simulink model "WG0920_3D"  (R2013a)
settings: Solver=ode3  StartTime=0.0  StopTime=T  FixedStep=dt  RelTol=1e-3
values from neighbouring files (symbols this model uses):
  dt = 1e-2    (= 0.01)    [WGSim.m]
  vi = [0,0,0,0,0,0,0,0,0,0,0,0]    [WGSim.m]
  xi = [0,0,0,0,0,0,0,0,0,0,0,0]    [WGSim.m]
libraries: simulink x2
settings Model: Creator=user  LastModifiedBy=user

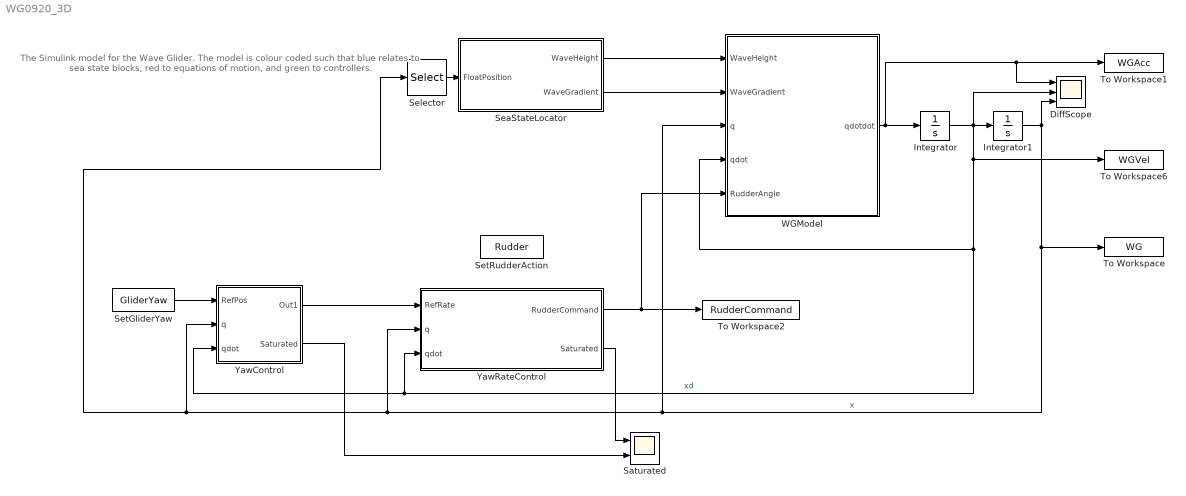
== system WG0920_3D ==
  note: The Simulink model for the Wave Glider.
      | The model is colour coded such that blue
      | relates to sea state blocks, red to equations
      | of motion, and green to controllers.
  DiffScope : Scope  NumInputPorts=3
      settings: ShowLegends=on  TimeRange=10  YMin=-17~-1.1~-2  YMax=5~0.8~4.5
  Integrator : Integrator  InitialCondition=vi  ContinuousStateAttributes='velocity'
  Integrator1 : Integrator  InitialCondition=xi  ContinuousStateAttributes='position'
  Saturated : Scope  NumInputPorts=2
      settings: ShowLegends=on  YMin=-2.75~-2  YMax=2~2  SaveName=ScopeData15
  SeaStateLocator : Subsystem
  Selector : Selector  InputPortWidth=12  IndexOptions=Index vector (dialog)  Indices=[1 2]  OutputSizes=1
  SetGliderYaw : FromWorkspace  VariableName=GliderYaw  SampleTime=0  OutputAfterFinalValue=Holding final value
  SetRudderAction : FromWorkspace  VariableName=Rudder  SampleTime=0  OutputAfterFinalValue=Holding final value
  To Workspace : ToWorkspace  VariableName=WG  SampleTime=-1
  To Workspace1 : ToWorkspace  VariableName=WGAcc  SampleTime=-1
  To Workspace2 : ToWorkspace  VariableName=RudderCommand  SampleTime=-1
  To Workspace6 : ToWorkspace  VariableName=WGVel  SampleTime=-1
  WGModel : Subsystem
  YawControl : Subsystem
  YawRateControl : Subsystem
  wires:
  Integrator/1 -> DiffScope/2, YawControl/3(qdot), YawRateControl/3(qdot), WGModel/4(qdot), To Workspace6/1, Integrator1/1  "xd"
  Integrator1/1 -> DiffScope/3, WGModel/3(q), YawRateControl/2(q), YawControl/2(q), Selector/1, To Workspace/1  "x"
  WGModel/1(qdotdot) -> DiffScope/1, To Workspace1/1, Integrator/1
  Selector/1 -> SeaStateLocator/1(FloatPosition)
  SeaStateLocator/1(WaveHeight) -> WGModel/1(WaveHeight)
  SeaStateLocator/2(WaveGradient) -> WGModel/2(WaveGradient)
  YawRateControl/1(RudderCommand) -> WGModel/5(RudderAngle), To Workspace2/1
  SetGliderYaw/1 -> YawControl/1(RefPos)
  YawControl/1(Out1) -> YawRateControl/1(RefRate)
  YawRateControl/2(Saturated) -> Saturated/1
  YawControl/2(Saturated) -> Saturated/2

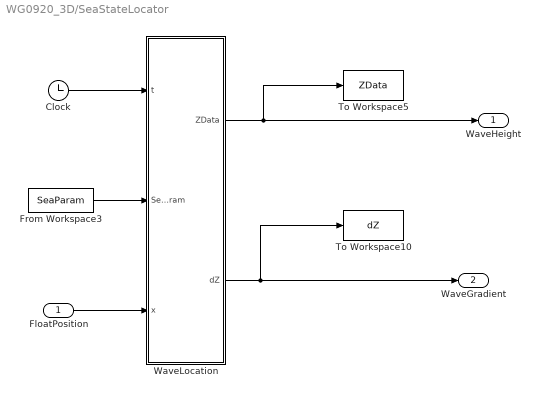
== system WG0920_3D/SeaStateLocator ==
  FloatPosition : Inport
  Clock : Clock
  From Workspace3 : FromWorkspace  VariableName=SeaParam  SampleTime=0  Interpolate=off  OutputAfterFinalValue=Holding final value
  To Workspace10 : ToWorkspace  VariableName=dZ  SampleTime=-1
  To Workspace5 : ToWorkspace  VariableName=ZData  SampleTime=-1
  WaveLocation : MATLAB Function  TreatAsAtomicUnit=on  SystemSampleTime=dt
  WaveHeight : Outport
  WaveGradient : Outport  Port=2
  wires:
  WaveLocation/1(ZData) -> WaveHeight/1, To Workspace5/1
  From Workspace3/1 -> WaveLocation/2(SeaParam)
  WaveLocation/2(dZ) -> To Workspace10/1, WaveGradient/1
  FloatPosition/1 -> WaveLocation/3(x)
  Clock/1 -> WaveLocation/1(t)

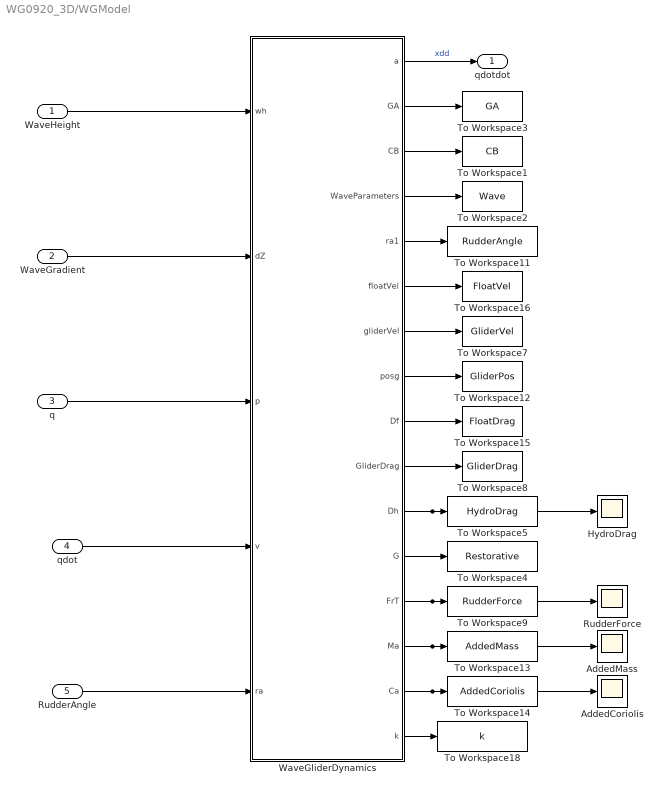
== system WG0920_3D/WGModel ==
  WaveHeight : Inport
  WaveGradient : Inport  Port=2
  q : Inport  Port=3
  qdot : Inport  Port=4
  RudderAngle : Inport  Port=5
  AddedCoriolis : Scope
      settings: ShowLegends=on  SaveName=ScopeData13
  AddedMass : Scope
      settings: ShowLegends=on  SaveName=ScopeData7
  HydroDrag : Scope
      settings: ShowLegends=on
  RudderForce : Scope
      settings: ShowLegends=on  SaveName=ScopeData9
  To Workspace1 : ToWorkspace  VariableName=CB  SampleTime=-1
  To Workspace11 : ToWorkspace  VariableName=RudderAngle  SampleTime=-1
  To Workspace12 : ToWorkspace  VariableName=GliderPos  SampleTime=-1
  To Workspace13 : ToWorkspace  VariableName=AddedMass  SampleTime=-1
  To Workspace14 : ToWorkspace  VariableName=AddedCoriolis  SampleTime=-1
  To Workspace15 : ToWorkspace  VariableName=FloatDrag  SampleTime=-1
  To Workspace16 : ToWorkspace  VariableName=FloatVel  SampleTime=-1
  To Workspace18 : ToWorkspace  VariableName=k  SampleTime=-1
  To Workspace2 : ToWorkspace  VariableName=Wave  SampleTime=-1
  To Workspace3 : ToWorkspace  VariableName=GA  SampleTime=-1
  To Workspace4 : ToWorkspace  VariableName=Restorative  SampleTime=-1
  To Workspace5 : ToWorkspace  VariableName=HydroDrag  SampleTime=-1
  To Workspace7 : ToWorkspace  VariableName=GliderVel  SampleTime=-1
  To Workspace8 : ToWorkspace  VariableName=GliderDrag  SampleTime=-1
  To Workspace9 : ToWorkspace  VariableName=RudderForce  SampleTime=-1
  WaveGliderDynamics : MATLAB Function  TreatAsAtomicUnit=on
  qdotdot : Outport
  wires:
  WaveGliderDynamics/12(G) -> To Workspace4/1
  WaveGliderDynamics/13(FrT) -> RudderForce/1, To Workspace9/1
  WaveGliderDynamics/4(WaveParameters) -> To Workspace2/1
  WaveGradient/1 -> WaveGliderDynamics/2(dZ)
  WaveGliderDynamics/1(a) -> qdotdot/1  "xdd"
  WaveGliderDynamics/10(GliderDrag) -> To Workspace8/1
  WaveGliderDynamics/16(k) -> To Workspace18/1
  WaveGliderDynamics/8(posg) -> To Workspace12/1
  WaveGliderDynamics/9(Df) -> To Workspace15/1
  WaveGliderDynamics/15(Ca) -> AddedCoriolis/1, To Workspace14/1
  WaveHeight/1 -> WaveGliderDynamics/1(wh)
  q/1 -> WaveGliderDynamics/3(p)
  qdot/1 -> WaveGliderDynamics/4(v)
  WaveGliderDynamics/3(CB) -> To Workspace1/1
  WaveGliderDynamics/5(ra1) -> To Workspace11/1
  WaveGliderDynamics/2(GA) -> To Workspace3/1
  RudderAngle/1 -> WaveGliderDynamics/5(ra)
  WaveGliderDynamics/6(floatVel) -> To Workspace16/1
  WaveGliderDynamics/14(Ma) -> AddedMass/1, To Workspace13/1
  WaveGliderDynamics/7(gliderVel) -> To Workspace7/1
  WaveGliderDynamics/11(Dh) -> To Workspace5/1, HydroDrag/1

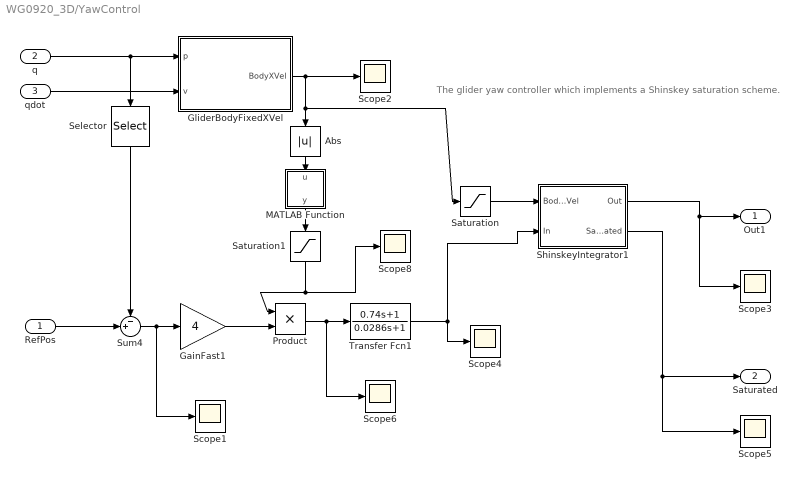
== system WG0920_3D/YawControl ==
  note: The glider yaw controller which implements
      | a Shinskey saturation scheme.
  RefPos : Inport
  q : Inport  Port=2
  qdot : Inport  Port=3
  Abs : Abs
  GainFast1 : Gain  Gain=4
  GliderBodyFixedXVel : MATLAB Function  TreatAsAtomicUnit=on
  MATLAB Function : MATLAB Function  TreatAsAtomicUnit=on
  Product : Product
  Saturation : Saturate  UpperLimit=1.5  LowerLimit=0.1
  Saturation1 : Saturate  UpperLimit=1  LowerLimit=0.01
  Scope{1..6,8} (7 alike) : Scope
      Scope1 settings: YMin=-0.45  YMax=0.2  SaveName=ScopeData10
      Scope2 settings: YMin=-0.2  YMax=0.2  SaveName=ScopeData11
      Scope3 settings: YMin=-0.08  YMax=0.08  SaveName=ScopeData6
      Scope4 settings: YMin=0.01  YMax=0.05  SaveName=ScopeData12
      Scope5 settings: YMin=-0.2  YMax=1.2  SaveName=ScopeData14
      Scope6 settings: YMin=-0.025  YMax=0.25  SaveName=ScopeData17
      Scope8 settings: YMin=-0.025  YMax=0.25  SaveName=ScopeData16
  Selector : Selector  InputPortWidth=12  IndexOptions=Index vector (dialog)  Indices=[11]  OutputSizes=1
  ShinskeyIntegrator1 : Subsystem
  Sum4 : Sum  Inputs=-+|
  Transfer Fcn1 : TransferFcn  Numerator=[0.74 1]  Denominator=[0.0286 1]
  Out1 : Outport
  Saturated : Outport  Port=2
  wires:
  RefPos/1 -> Sum4/2
  q/1 -> GliderBodyFixedXVel/1(p), Selector/1
  Selector/1 -> Sum4/1
  ShinskeyIntegrator1/1(Out) -> Out1/1, Scope3/1
  Transfer Fcn1/1 -> Scope4/1, ShinskeyIntegrator1/2(In)
  qdot/1 -> GliderBodyFixedXVel/2(v)
  Sum4/1 -> Scope1/1, GainFast1/1
  Saturation/1 -> ShinskeyIntegrator1/1(BodyFixedVel)
  ShinskeyIntegrator1/2(Saturated) -> Scope5/1, Saturated/1
  GliderBodyFixedXVel/1(BodyXVel) -> Scope2/1, Abs/1, Saturation/1
  Saturation1/1 -> Scope8/1, Product/1
  Abs/1 -> MATLAB Function/1(u)
  MATLAB Function/1(y) -> Saturation1/1
  GainFast1/1 -> Product/2
  Product/1 -> Transfer Fcn1/1, Scope6/1

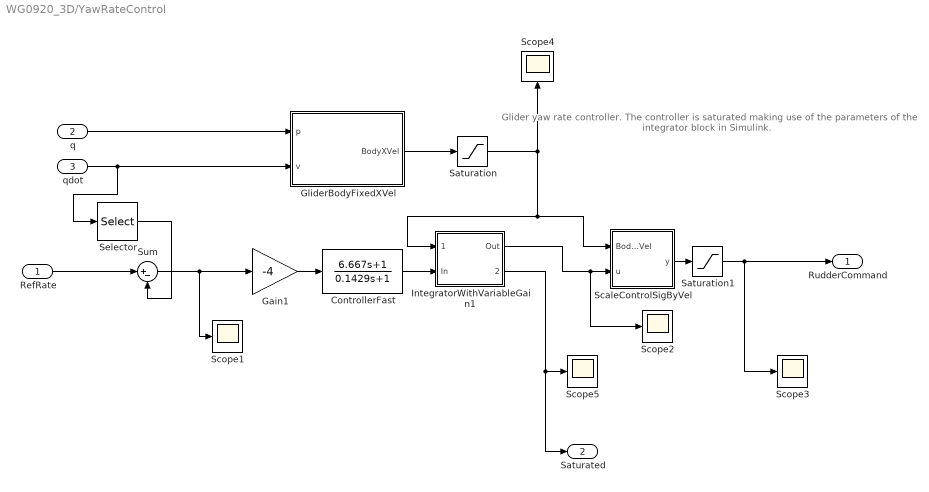
== system WG0920_3D/YawRateControl ==
  note: Glider yaw rate controller. The controller
      | is saturated making use of the parameters
      | of the integrator block in Simulink.
  RefRate : Inport
  q : Inport  Port=2
  qdot : Inport  Port=3
  ControllerFast : TransferFcn  Numerator=[6.667 1]  Denominator=[0.1429 1]
  Gain1 : Gain  Gain=-4
  GliderBodyFixedXVel : MATLAB Function  TreatAsAtomicUnit=on
  IntegratorWithVariableGain1 : Subsystem
  Saturation : Saturate  UpperLimit=1.5  LowerLimit=0.1
  Saturation1 : Saturate  UpperLimit=pi/18*5  LowerLimit=-pi/18*5
  ScaleControlSigByVel : MATLAB Function  TreatAsAtomicUnit=on
  Scope{1..5} (5 alike) : Scope
      Scope1 settings: SaveName=ScopeData3
      Scope2 settings: SaveName=ScopeData4
      Scope3 settings: YMin=0.0665  YMax=0.0681  SaveName=ScopeData5
      Scope4 settings: YMin=-0.00085  YMax=-0.0001  SaveName=ScopeData2
      Scope5 settings: SaveName=ScopeData8
  Selector : Selector  InputPortWidth=12  IndexOptions=Index vector (dialog)  Indices=[11]  OutputSizes=1
  Sum : Sum  Inputs=|+-
  RudderCommand : Outport
  Saturated : Outport  Port=2
  wires:
  ScaleControlSigByVel/1(y) -> Saturation1/1
  Saturation/1 -> ScaleControlSigByVel/1(BodyXVel), IntegratorWithVariableGain1/1(BodyXVel), Scope4/1
  RefRate/1 -> Sum/1
  Sum/1 -> Scope1/1, Gain1/1
  Saturation1/1 -> Scope3/1, RudderCommand/1
  q/1 -> GliderBodyFixedXVel/1(p)
  qdot/1 -> Selector/1, GliderBodyFixedXVel/2(v)
  Selector/1 -> Sum/2
  Gain1/1 -> ControllerFast/1
  GliderBodyFixedXVel/1(BodyXVel) -> Saturation/1
  IntegratorWithVariableGain1/1(Out) -> Scope2/1, ScaleControlSigByVel/2(u)
  ControllerFast/1 -> IntegratorWithVariableGain1/2(In)
  IntegratorWithVariableGain1/2(Saturated) -> Saturated/1, Scope5/1

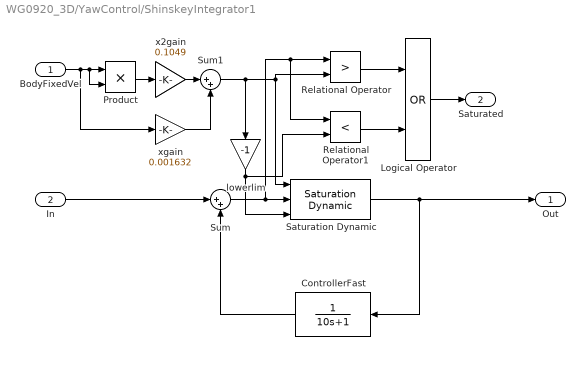
== system WG0920_3D/YawControl/ShinskeyIntegrator1 ==
  BodyFixedVel : Inport
  In : Inport  Port=2
  ControllerFast : TransferFcn  Denominator=[10 1]
  Logical Operator : Logic  Operator=OR  AllPortsSameDT=off  OutDataTypeStr=boolean
  Product : Product
  Relational Operator : RelationalOperator  Operator=>  OutDataTypeStr=boolean
  Relational Operator1 : RelationalOperator  Operator=<  OutDataTypeStr=boolean
  Saturation Dynamic : simulink/Discontinuities/Saturation Dynamic  OutMin=[]  OutMax=[]  OutDataTypeStr=Inherit: Same as second input  OutDataType=fixdt(1, 16)  OutScaling=2^-10  DoSatur=off
  Sum : Sum  Inputs=|++
  Sum1 : Sum  Inputs=|++
  lowerlim : Gain  Gain=-1
  x2gain : Gain  Gain=0.1049
  xgain : Gain  Gain=0.001632
  Out : Outport
  Saturated : Outport  Port=2
  wires:
  In/1 -> Sum/1
  Saturation Dynamic/1 -> ControllerFast/1, Out/1
  Sum/1 -> Relational Operator1/1, Relational Operator/1, Saturation Dynamic/2
  ControllerFast/1 -> Sum/2
  Sum1/1 -> Saturation Dynamic/1, Relational Operator/2, lowerlim/1
  lowerlim/1 -> Relational Operator1/2, Saturation Dynamic/3
  BodyFixedVel/1 -> xgain/1, Product/2, Product/1
  Product/1 -> x2gain/1
  x2gain/1 -> Sum1/1
  xgain/1 -> Sum1/2
  Relational Operator/1 -> Logical Operator/1
  Relational Operator1/1 -> Logical Operator/2
  Logical Operator/1 -> Saturated/1

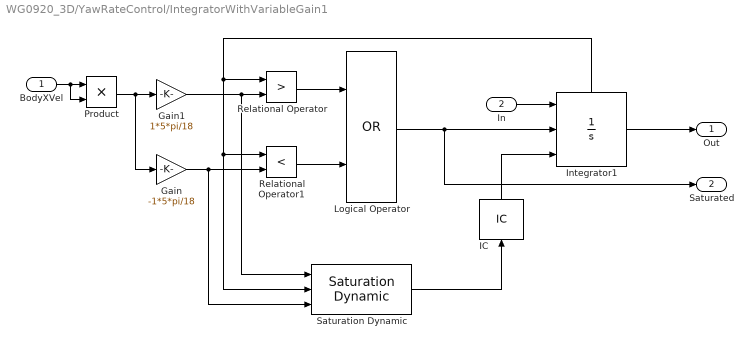
== system WG0920_3D/YawRateControl/IntegratorWithVariableGain1 ==
  BodyXVel : Inport
  In : Inport  Port=2
  Gain : Gain  Gain=-1*5*pi/18
  Gain1 : Gain  Gain=1*5*pi/18
  IC : InitialCondition  Value=0
  Integrator1 : Integrator  ExternalReset=level  InitialConditionSource=external  UpperSaturationLimit=5*pi/8  LowerSaturationLimit=-5*pi/8  ShowStatePort=on
  Logical Operator : Logic  Operator=OR  AllPortsSameDT=off  OutDataTypeStr=boolean
  Product : Product
  Relational Operator : RelationalOperator  Operator=>  OutDataTypeStr=boolean
  Relational Operator1 : RelationalOperator  Operator=<  OutDataTypeStr=boolean
  Saturation Dynamic : simulink/Discontinuities/Saturation Dynamic  OutMin=[]  OutMax=[]  OutDataTypeStr=Inherit: Same as second input  OutDataType=fixdt(1, 16)  OutScaling=2^-10  DoSatur=off
  Out : Outport
  Saturated : Outport  Port=2
  wires:
  Product/1 -> Gain1/1, Gain/1
  BodyXVel/1 -> Product/1, Product/2
  IC/1 -> Integrator1/3
  Saturation Dynamic/1 -> IC/1
  Logical Operator/1 -> Integrator1/2, Saturated/1
  Gain/1 -> Relational Operator1/2, Saturation Dynamic/3
  Gain1/1 -> Relational Operator/2, Saturation Dynamic/1
  Integrator1/State -> Relational Operator1/1, Saturation Dynamic/2, Relational Operator/1
  Relational Operator1/1 -> Logical Operator/2
  Relational Operator/1 -> Logical Operator/1
  Integrator1/1 -> Out/1
  In/1 -> Integrator1/1

== matlab function WG0920_3D/SeaStateLocator/WaveLocation ==
  data: t input; SeaParam input; ZData output; x input; dZ output
% Determine the sea parameters at the location of the Wave Glider model.
function [ZData, dZ]  = fcn(t,SeaParam,x)

% Sea parameters
numOfSignals = SeaParam(1);
amplitude = SeaParam(2:1+numOfSignals);
freq = SeaParam(2+numOfSignals:1+numOfSignals*2);
off = SeaParam(2+numOfSignals*2);
ang = SeaParam(3+numOfSignals*2)*pi/180;
g = 9.81;

% Location and angle
px = x(1);
py = x(2);
dir = [cos(ang) -sin(ang);sin(ang) cos(ang)]*[off;0];
xoff = dir(1);
yoff = dir(2);

% Instantiating sea parameters
ZData = 0;
dZdx = 0;
dZdy = 0;

R = sqrt((px-xoff).^2 + (py-yoff).^2);

for i = 1:numOfSignals
    w = freq(i);
    A = amplitude(i);
    T = 1/w;
    k = w^2/g;
    phi = t/T;
    ZData = ZData + A*sin(k*R-phi);
    dZdx = dZdx + A*k*(px-xoff)./R.*cos(k*R-phi);
	dZdy = dZdy + A*k*(py-yoff)./R.*cos(k*R-phi);
end

dZ = [dZdx;dZdy];

== matlab function WG0920_3D/WGModel/WaveGliderDynamics ==
  data: wh input; dZ input; a output; GA output; p input; v input; CB output; WaveParameters output; ra1 output; floatVel output; gliderVel output; posg output; Df output; GliderDrag output; Dh output; G output; FrT output; Ma output; ra input; Ca output; k output
% Function block that determines equations of motions for the Wave Glider
% model. The rigid-body EOM are determines based on functions generated in
% the createEquations function. The hydrostatic forces on the glider are
% assumed constant based on the position of the glider, while the float
% parameters are calculated based on the generalised coordinates. The added
% mass is calculated based on the functions generated in the
% createEquations function.
function [a,GA,CB,WaveParameters,ra1,floatVel,gliderVel,posg,Df,GliderDrag,Dh,G,FrT,Ma,Ca,k] = fcn(wh,dZ,p,v,ra)

% Constants
g = 9.81;
rho = 1000;
floatHeight = 0.23;

% Input Wave Properties
WaveParameters = [wh;dZ];
dZdx = dZ(1);
dZdy = dZ(2);

% Rudder Angle
ra1 = ra;

% Variable assignment
xf = p(1);
yf = p(2);
zf = p(3);
phif = p(4);
thetaf = p(5);
psif = p(6);
phit = p(7);
thetat = p(8);
phig = p(9);
thetag = p(10);
psig = p(11);
thetaa = p(12);
dxf = v(1);
dyf = v(2);
dzf = v(3);
dphif = v(4);
dthetaf = v(5);
dpsif = v(6);
dphit = v(7);
dthetat = v(8);
dphig = v(9);
dthetag = v(10);
dpsig = v(11);
dthetaa = v(12);

M = get_M2017_06_10(p,v);
C11 = get_C112017_06_10(p,v);
C12 = get_C122017_06_10(p,v);
C13 = get_C132017_06_10(p,v);
C21 = get_C212017_06_10(p,v);
C22 = get_C222017_06_10(p,v);
C23 = get_C232017_06_10(p,v);
C31 = get_C312017_06_10(p,v);
C32 = get_C322017_06_10(p,v);
C33 = get_C332017_06_10(p,v);
C = [C11,C12,C13;
     C21,C22,C23;
     C31,C32,C33];

D = get_D2017_06_10(p,v);
sl = get_sl2017_06_10(p,v);
k = getSpringConstant(sl,thetaa,thetag);

% Buoyancy calculation
% Glider
posg = get_pg2017_06_10(p,v);
if(posg(3)>wh)
    fBg = 0.0187*g*rho;
    CBxg = 0;
    CByg = 0;
    CBzg = 0;
    Gg = get_QGenGlider(p,v,[0;0;fBg],[CBxg;CByg;CBzg]); 
else
    Gg = zeros(size(p));
end
% Float
vol = 0;
CB = [0;0;0];
coder.extrinsic('FloatBuoy');
[vol,CB] = FloatBuoy(p,[dZ;wh]);
fB = vol*g*rho;
Bf = [0;0;fB];                
Gf = get_QGenFloat(p,v,Bf,CB);
G = get_G2017_06_10(p,v,k);
G = G + Gf + Gg;

% Glider drag,force and position
Rgx = [1,0,0;
       0,cos(phig),-sin(phig);
       0,sin(phig),cos(phig)];
Rgy = [cos(thetag),0,sin(thetag);
    0,1,0;
     -sin(thetag),0,cos(thetag)];
Rgz = [cos(psig),-sin(psig),0;
       sin(psig),cos(psig),0;
       0,0,1];
Rg = Rgx*Rgy*Rgz;
velG = get_dpg2017_06_10(p,v);
vgb = Rg'*velG;
gliderVel = [velG;vgb];
if vgb(3)>=0
    GA = 1;
else
    GA = 0;
end
[Dlg,Dag] = DragGlider(v,vgb);
Fb = Dlg*[1;1;1;1;1;1];
Fi = Rg*Fb;
GliderDrag = getGenForce(p,v,Fi,zeros(9,1),3);
GliderAngDrag = Dag*[1;1;1;1;1;1];
GliderDrag(9:11) = GliderDrag(9:11) + GliderAngDrag;

%Float drag
Rfx = [1,0,0;
       0,cos(phif),-sin(phif);
       0,sin(phif),cos(phif)];
Rfy = [cos(thetaf),0,sin(thetaf);
       0,1,0;
       -sin(thetaf),0,cos(thetaf)];
Rfz = [cos(psif),-sin(psif),0;
       sin(psif),cos(psif),0;
       0,0,1];
Rf = Rfz*Rfy*Rfx;
velF = get_dpf2017_06_10(p,v);
vfb = Rf.'*velF;
floatVel = [velF;vfb];
if ((zf-wh)>-floatHeight/2)          % Toggle hydrodynamics on float
    floatHydro = 1;
    [Dfl,Dfa] = DragFloat(v,vfb);
    Dfb = Dfl*[1;1;1;1;1;1];
    Dfi = Rf*Dfb;
    Df = getGenForce(p,v,Dfi,zeros(9,1),1);
    Df(4:6) = Df(4:6) + Dfa*[1;1;1;1;1;1];
else
    floatHydro = 0;
    Df = zeros(12,1);
end

% Rudder Forces
Fr = RudderForce(vgb(1),ra1);
Fr(1:3) = Rg*Fr(1:3);
FrL = getGenForce(p,v,Fr(1:3),zeros(9,1),3);
FrT = FrL + [zeros(8,1);Fr(4:6);zeros(1,1)];

% Added Mass
[Ma,Ca] = AddedMass(p,v,vfb,vgb,floatHydro);

% Hydrofoil Forces
Hf = HydrofoilForce(vgb(1),vgb(3),(thetaa-thetag),v);
Hfi = Rg*[Hf(1);0;Hf(2)];
Dh = getGenForce(p,v,Hfi,zeros(9,1),3) + [zeros(11,1);Hf(3)];

% Drag consolidation
Q = GliderDrag + Df + Dh;

% Changes


% Output accelerations
a = (M + Ma)\(-C*v - Ca*v - G - [0;0;0;0;0;0;1;1;0;0;0;0].*(D*v) + Q + FrT);

== matlab function WG0920_3D/YawRateControl/ScaleControlSigByVel ==
  data: BodyXVel input; u input; y output
function y = fcn(BodyXVel,u)
%#codegen

y = u/(BodyXVel^2);

== matlab function WG0920_3D/YawRateControl/GliderBodyFixedXVel ==
  data: p input; v input; BodyXVel output
% Determining the body-fixed x velocity of the glider based on the
% generalised coordinates.
function BodyXVel = fcn(p,v)
%#codegen

phig = p(9);
thetag = p(10);
psig = p(11);

Rgx = [1,0,0;
       0,cos(phig),-sin(phig);
       0,sin(phig),cos(phig)];
Rgy = [cos(thetag),0,sin(thetag);
    0,1,0;
     -sin(thetag),0,cos(thetag)];
Rgz = [cos(psig),-sin(psig),0;
       sin(psig),cos(psig),0;
       0,0,1];
Rg = Rgx*Rgy*Rgz;
velG = get_dpg2017_09_21(p,v);
vgb = Rg'*velG;

BodyXVel = vgb(1);

== matlab function WG0920_3D/YawControl/GliderBodyFixedXVel ==
  data: p input; v input; BodyXVel output
% Determining the body-fixed x velocity of the glider based on the
% generalised coordinates.
function BodyXVel = fcn(p,v)
%#codegen

phig = p(9);
thetag = p(10);
psig = p(11);

Rgx = [1,0,0;
       0,cos(phig),-sin(phig);
       0,sin(phig),cos(phig)];
Rgy = [cos(thetag),0,sin(thetag);
    0,1,0;
     -sin(thetag),0,cos(thetag)];
Rgz = [cos(psig),-sin(psig),0;
       sin(psig),cos(psig),0;
       0,0,1];
Rg = Rgx*Rgy*Rgz;
velG = get_dpg2017_09_21(p,v);
vgb = Rg'*velG;

BodyXVel = vgb(1);

== matlab function WG0920_3D/YawControl/MATLAB Function ==
  data: u input; y output
function y = fcn(u)
%#codegen

y = u;
